simulink library "inp"  (R2021b)
settings: Solver=VariableStepAuto  StartTime=0.0  StopTime=10.0  RelTol=1e-3
undefined symbols (not defined in the file): C_TASK_5MS_S, FALSE, KINP_AcoreReadyToSlp_flg_ovrdflg, KINP_AcoreReadyToSlp_flg_ovrdval, KINP_AllowMovThd_OTA_enum_ovrdflg, KINP_AllowMovThd_OTA_enum_ovrdval, KINP_APSAngleTarget_Deg_ovrdflg, KINP_APSAngleTarget_Deg_ovrdval, KINP_APSDecReq_mps2_ovrdflg, KINP_APSDecReq_mps2_ovrdval, KINP_APSDecReqA_flg_ovrdflg, KINP_APSDecReqA_flg_ovrdval, KINP_APSDFLL_cm_ovrdflg, KINP_APSDFLL_cm_ovrdval, KINP_APSDFLR_cm_ovrdflg, KINP_APSDFLR_cm_ovrdval, KINP_APSDRLL_cm_ovrdflg, KINP_APSDRLL_cm_ovrdval, KINP_APSDRLR_cm_ovrdflg, KINP_APSDRLR_cm_ovrdval, KINP_APSExitCondition_enum_ovrdflg, KINP_APSExitCondition_enum_ovrdval, KINP_APSHWVer_enum_ovrdflg, KINP_APSHWVer_enum_ovrdval, KINP_APSProgressPCT_pct_ovrdflg, KINP_APSProgressPCT_pct_ovrdval, KINP_APSReq_enum_ovrdflg, KINP_APSReq_enum_ovrdval, KINP_APSRQDisplay_enum_ovrdflg, KINP_APSRQDisplay_enum_ovrdval, KINP_APSRqEPASCtrl_flg_ovrdflg, KINP_APSRqEPASCtrl_flg_ovrdval, KINP_APSShiftPosnReq_enum_ovrdval, KINP_APSShiftPosnReq_enum_ovrflg, KINP_APSSpeedCMD_kph_ovrdval, KINP_APSSpeedCMD_kph_ovrflg, KINP_APSStaSystem_enum_ovrdflg, KINP_APSStaSystem_enum_ovrdval, KINP_APSSWVer_enum_ovrdflg, KINP_APSSWVer_enum_ovrdval, KINP_APSVMCReqA_flg_ovrdval, KINP_APSVMCReqA_flg_ovrflg, KINP_APSVRqEPASCtrl_flg_ovrdflg, KINP_APSVRqEPASCtrl_flg_ovrdval, KINP_AuxBattVolmV_mV_ovrdflg, KINP_AuxBattVolmV_mV_ovrdval, KINP_CAASSta_enum_ovrdflg, KINP_CAASSta_enum_ovrdval, KINP_CAASVMCReqA_flg_ovrdval, KINP_CAASVMCReqA_flg_ovrflg, KINP_Chime_enum_ovrdflg, KINP_Chime_enum_ovrdval, KINP_ClearDTCcmd_flg_ovrdflg, KINP_ClearDTCcmd_flg_ovrdval, KINP_EvccAplusPwrUpReq_flg_ovrdflg, KINP_EvccAplusPwrUpReq_flg_ovrdval, KINP_LFID_raw_ovrdval, KINP_LFID_raw_ovrflg, KINP_LRID_raw_ovrdval, KINP_MemOffsetAccX_raw16_ovrdflg ... (+118)
libraries: FVT_lib x503, hcu_lib x1
(part 3 of 16)

== system inp/INP/CAN1/CommunicationCheck ==
  BHAL_outputs : Inport
  CANMsgInvalidDCDCStatus1 : FVT_lib/inp/CAN_Msg_Validity_Process_template  SystemSampleTime=-1  VariantActivationTime=update diagram  Latency=0  AutoFrameSizeCalculation=off
      link override ovrdflg: Value=KINP_CANMsgInvalidDCDCStatus1_flg_ovrdflg
      link override ovrdval: Value=KINP_CANMsgInvalidDCDCStatus1_flg_ovrdval
  CANMsgInvalidDCDCStatus2 : FVT_lib/inp/CAN_Msg_Validity_Process_template  SystemSampleTime=-1  VariantActivationTime=update diagram  Latency=0  AutoFrameSizeCalculation=off
      link override ovrdflg: Value=KINP_CANMsgInvalidDCDCStatus2_flg_ovrdflg
      link override ovrdval: Value=KINP_CANMsgInvalidDCDCStatus2_flg_ovrdval
  CANMsgInvalidEACStatus1 : FVT_lib/inp/CAN_Msg_Validity_Process_template  SystemSampleTime=-1  VariantActivationTime=update diagram  Latency=0  AutoFrameSizeCalculation=off
      link override ovrdflg: Value=KINP_CANMsgInvalidEACStatus1_flg_ovrdflg
      link override ovrdval: Value=KINP_CANMsgInvalidEACStatus1_flg_ovrdval
  CANMsgInvalidEBC1 : FVT_lib/inp/CAN_Msg_Validity_Process_template  SystemSampleTime=-1  VariantActivationTime=update diagram  Latency=0  AutoFrameSizeCalculation=off
      link override ovrdflg: Value=KINP_CANMsgInvalidEBC1_flg_ovrdflg
      link override ovrdval: Value=KINP_CANMsgInvalidEBC1_flg_ovrdval
  CANMsgInvalidEBC2 : FVT_lib/inp/CAN_Msg_Validity_Process_template  SystemSampleTime=-1  VariantActivationTime=update diagram  Latency=0  AutoFrameSizeCalculation=off
      link override ovrdflg: Value=KINP_CANMsgInvalidEBC2_flg_ovrdflg
      link override ovrdval: Value=KINP_CANMsgInvalidEBC2_flg_ovrdval
  CANMsgInvalidEBC5 : FVT_lib/inp/CAN_Msg_Validity_Process_template  SystemSampleTime=-1  VariantActivationTime=update diagram  Latency=0  AutoFrameSizeCalculation=off
      link override ovrdflg: Value=KINP_CANMsgInvalidEBC5_flg_ovrdflg
      link override ovrdval: Value=KINP_CANMsgInvalidEBC5_flg_ovrdval
  CANMsgInvalidEHPSStatus1 : FVT_lib/inp/CAN_Msg_Validity_Process_template  SystemSampleTime=-1  VariantActivationTime=update diagram  Latency=0  AutoFrameSizeCalculation=off
      link override ovrdflg: Value=KINP_CANMsgInvalidEHPSStatus1_flg_ovrdflg
      link override ovrdval: Value=KINP_CANMsgInvalidEHPSStatus1_flg_ovrdval
  CANMsgInvalidEMC1EM1 : FVT_lib/inp/CAN_Msg_Validity_Process_template  SystemSampleTime=-1  VariantActivationTime=update diagram  Latency=0  AutoFrameSizeCalculation=off
      link override ovrdflg: Value=KINP_CANMsgInvalidEMC1EM1_flg_ovrdflg
      link override ovrdval: Value=KINP_CANMsgInvalidEMC1EM1_flg_ovrdval
  CANMsgInvalidEPB1 : FVT_lib/inp/CAN_Msg_Validity_Process_template  SystemSampleTime=-1  VariantActivationTime=update diagram  Latency=0  AutoFrameSizeCalculation=off
      link override ovrdflg: Value=KINP_CANMsgInvalidEPB1_flg_ovrdflg
      link override ovrdval: Value=KINP_CANMsgInvalidEPB1_flg_ovrdval
  CANMsgInvalidPDUStatus1 : FVT_lib/inp/CAN_Msg_Validity_Process_template  SystemSampleTime=-1  VariantActivationTime=update diagram  Latency=0  AutoFrameSizeCalculation=off
      link override ovrdflg: Value=KINP_CANMsgInvalidPDUStatus1_flg_ovrdflg
      link override ovrdval: Value=KINP_CANMsgInvalidPDUStatus1_flg_ovrdval
  bus_creator : BusCreator  Inputs=10
  bus_selector : BusSelector  OutputSignals=VHAL_CANMsgInvalidDCDCStatus1_flg,VHAL_CANMsgInvalidDCDCStatus2_flg,VHAL_CANMsgInvalidEACStatus1_flg,VHAL_CANMsgInvalidEBC1_flg,VHAL_CANMsgInvalidEBC2_flg,VHAL_CANMsgInvalidEBC5_flg,VHAL_CANMsgInvalidEHPSStatus1_flg,VHAL_CANMsgInvalidEMC1EM1_flg,VHAL_CANMsgInvalidEPB1_flg,VHAL_CANMsgInvalidPDUStatus1_flg
  not{1..10} (10 alike) : Logic  Operator=NOT  AllPortsSameDT=off  OutDataTypeStr=boolean
  inp_CanValid_bus : Outport
  wires:
  BHAL_outputs/1 -> [BHAL_outputs]
  bus_selector/1 -> CANMsgInvalidDCDCStatus1/1  "<VHAL_CANMsgInvalidDCDCStatus1_flg>"
  CANMsgInvalidDCDCStatus1/1 -> not1/1
  not1/1 -> bus_creator/1  "VINP_CANMsgValidDCDCStatus1_flg"
  bus_selector/2 -> CANMsgInvalidDCDCStatus2/1  "<VHAL_CANMsgInvalidDCDCStatus2_flg>"
  CANMsgInvalidDCDCStatus2/1 -> not2/1
  not2/1 -> bus_creator/2  "VINP_CANMsgValidDCDCStatus2_flg"
  bus_selector/3 -> CANMsgInvalidEACStatus1/1  "<VHAL_CANMsgInvalidEACStatus1_flg>"
  CANMsgInvalidEACStatus1/1 -> not3/1
  not3/1 -> bus_creator/3  "VINP_CANMsgValidEACStatus1_flg"
  bus_selector/4 -> CANMsgInvalidEBC1/1  "<VHAL_CANMsgInvalidEBC1_flg>"
  CANMsgInvalidEBC1/1 -> not4/1
  not4/1 -> bus_creator/4  "VINP_CANMsgValidEBC1_flg"
  bus_selector/5 -> CANMsgInvalidEBC2/1  "<VHAL_CANMsgInvalidEBC2_flg>"
  CANMsgInvalidEBC2/1 -> not5/1
  not5/1 -> bus_creator/5  "VINP_CANMsgValidEBC2_flg"
  bus_selector/6 -> CANMsgInvalidEBC5/1  "<VHAL_CANMsgInvalidEBC5_flg>"
  CANMsgInvalidEBC5/1 -> not6/1
  not6/1 -> bus_creator/6  "VINP_CANMsgValidEBC5_flg"
  bus_selector/7 -> CANMsgInvalidEHPSStatus1/1  "<VHAL_CANMsgInvalidEHPSStatus1_flg>"
  CANMsgInvalidEHPSStatus1/1 -> not7/1
  not7/1 -> bus_creator/7  "VINP_CANMsgValidEHPSStatus1_flg"
  bus_selector/8 -> CANMsgInvalidEMC1EM1/1  "<VHAL_CANMsgInvalidEMC1EM1_flg>"
  CANMsgInvalidEMC1EM1/1 -> not8/1
  not8/1 -> bus_creator/8  "VINP_CANMsgValidEMC1EM1_flg"
  bus_selector/9 -> CANMsgInvalidEPB1/1  "<VHAL_CANMsgInvalidEPB1_flg>"
  CANMsgInvalidEPB1/1 -> not9/1
  not9/1 -> bus_creator/9  "VINP_CANMsgValidEPB1_flg"
  bus_selector/10 -> CANMsgInvalidPDUStatus1/1  "<VHAL_CANMsgInvalidPDUStatus1_flg>"
  CANMsgInvalidPDUStatus1/1 -> not10/1
  not10/1 -> bus_creator/10  "VINP_CANMsgValidPDUStatus1_flg"
  [BHAL_outputs] -> bus_selector/1
  bus_creator/1 -> inp_CanValid_bus/1

== system inp/INP/CAN1/CreateBus ==
  inp_CanValid_bus : Inport
  inp_Hal_bus : Inport  Port=2
  UnitConverter_{1..10} (10 alike) : DataTypeConversion  OutDataTypeStr=boolean
  UnitConverter_{11,13..22,24..28,30..31,33..35,39..43,45..53,58..62} (40 alike) : DataTypeConversion  OutDataTypeStr=uint8
  UnitConverter_{12,23,29,32,36..38,44,54..57} (12 alike) : DataTypeConversion  OutDataTypeStr=single
  bus_creator : BusCreator  Inputs=62
  bus_selector : BusSelector  OutputSignals=VINP_CANMsgValidDCDCStatus1_flg,VINP_CANMsgValidDCDCStatus2_flg,VINP_CANMsgValidEACStatus1_flg,VINP_CANMsgValidEBC1_flg,VINP_CANMsgValidEBC2_flg,VINP_CANMsgValidEBC5_flg,VINP_CANMsgValidEHPSStatus1_flg,VINP_CANMsgValidEMC1EM1_flg,VINP_CANMsgValidEPB1_flg,VINP_CANMsgValidPDUStatus1_flg
  bus_selector_1 : BusSelector  OutputSignals=VINP_DCDCEnSta_enum,VINP_DCDCOutVol_V,VINP_EACEnSta_enum,VINP_ABSFullyOper_enum,VINP_ABSOffroadSw_enum,VINP_ASRBrakeCtrlAtc_enum,VINP_ASREngCtrlAtc_enum,VINP_ASRHillHolderSw_enum,VINP_ASROffroadSw_enum,VINP_ATCASRInfoSig_enum,VINP_AcltrInterlockSw_enum,VINP_AntiLBrakABSAct_enum,VINP_BrakePedalPos_pct,VINP_EBSAmWarnLampSta_enum,VINP_EBSBrakeSw_enum,VINP_EBSRedWarnLampSta_enum,VINP_EngAuxShutdownSw_enum,VINP_EngDerateSw_enum,VINP_EngRetSel_pct,VINP_HaltBrakeSw_enum,VINP_RmAccelEnSw_enum,VINP_SACtrlBrakeCtrl_SA,VINP_TractCtrlOvrSw_enum,VINP_TrailerABSSta_enum,VINP_TrailerABSWarnSig_enum,VINP_FASpeed_kph,VINP_RelaSpdFALWheel_kph,VINP_RelaSpdFARWheel_kph,VINP_BrkTempeWarn_enum,VINP_FndBrkUse_enum,VINP_HaltBrkMode_enum,VINP_HillHolderMode_enum,VINP_ParkBrkActuFAct_enum,VINP_XBRAcltnLimit_mps2,VINP_XBRActtrlMode_enum,VINP_XBRSysSta_enum,VINP_EHPSEnSta_enum,VINP_EM1CS_enum,VINP_EM1Cnt_enum,VINP_EM1OvrCtrlMBrk_enum,VINP_EM1OvrCtrlMDriv_enum,VINP_EM1OvrCtrlMPriBrk_enum,VINP_EM1OvrCtrlMPriDriv_enum,VINP_EM1ReqTorqHRlsBrk_pct,VINP_EM1ReqTorqHRlsDri_pct,VINP_EM1ReqTorqLimBrk_pct,VINP_EM1ReqTorqLimDriv_pct,VINP_EPBParkingBrakeSta_enum,VINP_PDUDCDCRlySta_enum,VINP_PDUEACRlySta_enum,VINP_PDUEHPSRlySta_enum,VINP_PDUSelfChkSta_enum
  BINP_outputs : Outport
  wires:
  inp_CanValid_bus/1 -> [inp_CanValid_bus]
  inp_Hal_bus/1 -> [inp_Hal_bus]
  bus_selector/1 -> UnitConverter_1/1  "<VINP_CANMsgValidDCDCStatus1_flg>"
  UnitConverter_1/1 -> bus_creator/1  "VINP_CANMsgValidDCDCStatus1_flg"
  bus_selector/2 -> UnitConverter_2/1  "<VINP_CANMsgValidDCDCStatus2_flg>"
  UnitConverter_2/1 -> bus_creator/2  "VINP_CANMsgValidDCDCStatus2_flg"
  bus_selector/3 -> UnitConverter_3/1  "<VINP_CANMsgValidEACStatus1_flg>"
  UnitConverter_3/1 -> bus_creator/3  "VINP_CANMsgValidEACStatus1_flg"
  bus_selector/4 -> UnitConverter_4/1  "<VINP_CANMsgValidEBC1_flg>"
  UnitConverter_4/1 -> bus_creator/4  "VINP_CANMsgValidEBC1_flg"
  bus_selector/5 -> UnitConverter_5/1  "<VINP_CANMsgValidEBC2_flg>"
  UnitConverter_5/1 -> bus_creator/5  "VINP_CANMsgValidEBC2_flg"
  bus_selector/6 -> UnitConverter_6/1  "<VINP_CANMsgValidEBC5_flg>"
  UnitConverter_6/1 -> bus_creator/6  "VINP_CANMsgValidEBC5_flg"
  bus_selector/7 -> UnitConverter_7/1  "<VINP_CANMsgValidEHPSStatus1_flg>"
  UnitConverter_7/1 -> bus_creator/7  "VINP_CANMsgValidEHPSStatus1_flg"
  bus_selector/8 -> UnitConverter_8/1  "<VINP_CANMsgValidEMC1EM1_flg>"
  UnitConverter_8/1 -> bus_creator/8  "VINP_CANMsgValidEMC1EM1_flg"
  bus_selector/9 -> UnitConverter_9/1  "<VINP_CANMsgValidEPB1_flg>"
  UnitConverter_9/1 -> bus_creator/9  "VINP_CANMsgValidEPB1_flg"
  bus_selector/10 -> UnitConverter_10/1  "<VINP_CANMsgValidPDUStatus1_flg>"
  UnitConverter_10/1 -> bus_creator/10  "VINP_CANMsgValidPDUStatus1_flg"
  bus_selector_1/1 -> UnitConverter_11/1  "<VINP_DCDCEnSta_enum>"
  UnitConverter_11/1 -> bus_creator/11  "VINP_DCDCEnSta_enum"
  bus_selector_1/2 -> UnitConverter_12/1  "<VINP_DCDCOutVol_V>"
  UnitConverter_12/1 -> bus_creator/12  "VINP_DCDCOutVol_V"
  bus_selector_1/3 -> UnitConverter_13/1  "<VINP_EACEnSta_enum>"
  UnitConverter_13/1 -> bus_creator/13  "VINP_EACEnSta_enum"
  bus_selector_1/4 -> UnitConverter_14/1  "<VINP_ABSFullyOper_enum>"
  UnitConverter_14/1 -> bus_creator/14  "VINP_ABSFullyOper_enum"
  bus_selector_1/5 -> UnitConverter_15/1  "<VINP_ABSOffroadSw_enum>"
  UnitConverter_15/1 -> bus_creator/15  "VINP_ABSOffroadSw_enum"
  bus_selector_1/6 -> UnitConverter_16/1  "<VINP_ASRBrakeCtrlAtc_enum>"
  UnitConverter_16/1 -> bus_creator/16  "VINP_ASRBrakeCtrlAtc_enum"
  bus_selector_1/7 -> UnitConverter_17/1  "<VINP_ASREngCtrlAtc_enum>"
  UnitConverter_17/1 -> bus_creator/17  "VINP_ASREngCtrlAtc_enum"
  bus_selector_1/8 -> UnitConverter_18/1  "<VINP_ASRHillHolderSw_enum>"
  UnitConverter_18/1 -> bus_creator/18  "VINP_ASRHillHolderSw_enum"
  bus_selector_1/9 -> UnitConverter_19/1  "<VINP_ASROffroadSw_enum>"
  UnitConverter_19/1 -> bus_creator/19  "VINP_ASROffroadSw_enum"
  bus_selector_1/10 -> UnitConverter_20/1  "<VINP_ATCASRInfoSig_enum>"
  UnitConverter_20/1 -> bus_creator/20  "VINP_ATCASRInfoSig_enum"
  bus_selector_1/11 -> UnitConverter_21/1  "<VINP_AcltrInterlockSw_enum>"
  UnitConverter_21/1 -> bus_creator/21  "VINP_AcltrInterlockSw_enum"
  bus_selector_1/12 -> UnitConverter_22/1  "<VINP_AntiLBrakABSAct_enum>"
  UnitConverter_22/1 -> bus_creator/22  "VINP_AntiLBrakABSAct_enum"
  bus_selector_1/13 -> UnitConverter_23/1  "<VINP_BrakePedalPos_pct>"
  UnitConverter_23/1 -> bus_creator/23  "VINP_BrakePedalPos_pct"
  bus_selector_1/14 -> UnitConverter_24/1  "<VINP_EBSAmWarnLampSta_enum>"
  UnitConverter_24/1 -> bus_creator/24  "VINP_EBSAmWarnLampSta_enum"
  bus_selector_1/15 -> UnitConverter_25/1  "<VINP_EBSBrakeSw_enum>"
  UnitConverter_25/1 -> bus_creator/25  "VINP_EBSBrakeSw_enum"
  bus_selector_1/16 -> UnitConverter_26/1  "<VINP_EBSRedWarnLampSta_enum>"
  UnitConverter_26/1 -> bus_creator/26  "VINP_EBSRedWarnLampSta_enum"
  bus_selector_1/17 -> UnitConverter_27/1  "<VINP_EngAuxShutdownSw_enum>"
  UnitConverter_27/1 -> bus_creator/27  "VINP_EngAuxShutdownSw_enum"
  bus_selector_1/18 -> UnitConverter_28/1  "<VINP_EngDerateSw_enum>"
  UnitConverter_28/1 -> bus_creator/28  "VINP_EngDerateSw_enum"
  bus_selector_1/19 -> UnitConverter_29/1  "<VINP_EngRetSel_pct>"
  UnitConverter_29/1 -> bus_creator/29  "VINP_EngRetSel_pct"
  bus_selector_1/20 -> UnitConverter_30/1  "<VINP_HaltBrakeSw_enum>"
  UnitConverter_30/1 -> bus_creator/30  "VINP_HaltBrakeSw_enum"
  bus_selector_1/21 -> UnitConverter_31/1  "<VINP_RmAccelEnSw_enum>"
  UnitConverter_31/1 -> bus_creator/31  "VINP_RmAccelEnSw_enum"
  bus_selector_1/22 -> UnitConverter_32/1  "<VINP_SACtrlBrakeCtrl_SA>"
  UnitConverter_32/1 -> bus_creator/32  "VINP_SACtrlBrakeCtrl_SA"
  bus_selector_1/23 -> UnitConverter_33/1  "<VINP_TractCtrlOvrSw_enum>"
  UnitConverter_33/1 -> bus_creator/33  "VINP_TractCtrlOvrSw_enum"
  bus_selector_1/24 -> UnitConverter_34/1  "<VINP_TrailerABSSta_enum>"
  UnitConverter_34/1 -> bus_creator/34  "VINP_TrailerABSSta_enum"
  bus_selector_1/25 -> UnitConverter_35/1  "<VINP_TrailerABSWarnSig_enum>"
  UnitConverter_35/1 -> bus_creator/35  "VINP_TrailerABSWarnSig_enum"
  bus_selector_1/26 -> UnitConverter_36/1  "<VINP_FASpeed_kph>"
  UnitConverter_36/1 -> bus_creator/36  "VINP_FASpeed_kph"
  bus_selector_1/27 -> UnitConverter_37/1  "<VINP_RelaSpdFALWheel_kph>"
  UnitConverter_37/1 -> bus_creator/37  "VINP_RelaSpdFALWheel_kph"
  bus_selector_1/28 -> UnitConverter_38/1  "<VINP_RelaSpdFARWheel_kph>"
  UnitConverter_38/1 -> bus_creator/38  "VINP_RelaSpdFARWheel_kph"
  bus_selector_1/29 -> UnitConverter_39/1  "<VINP_BrkTempeWarn_enum>"
  UnitConverter_39/1 -> bus_creator/39  "VINP_BrkTempeWarn_enum"
  bus_selector_1/30 -> UnitConverter_40/1  "<VINP_FndBrkUse_enum>"
  UnitConverter_40/1 -> bus_creator/40  "VINP_FndBrkUse_enum"
  bus_selector_1/31 -> UnitConverter_41/1  "<VINP_HaltBrkMode_enum>"
  UnitConverter_41/1 -> bus_creator/41  "VINP_HaltBrkMode_enum"
  bus_selector_1/32 -> UnitConverter_42/1  "<VINP_HillHolderMode_enum>"
  UnitConverter_42/1 -> bus_creator/42  "VINP_HillHolderMode_enum"
  bus_selector_1/33 -> UnitConverter_43/1  "<VINP_ParkBrkActuFAct_enum>"
  UnitConverter_43/1 -> bus_creator/43  "VINP_ParkBrkActuFAct_enum"
  bus_selector_1/34 -> UnitConverter_44/1  "<VINP_XBRAcltnLimit_mps2>"
  UnitConverter_44/1 -> bus_creator/44  "VINP_XBRAcltnLimit_mps2"
  bus_selector_1/35 -> UnitConverter_45/1  "<VINP_XBRActtrlMode_enum>"
  UnitConverter_45/1 -> bus_creator/45  "VINP_XBRActtrlMode_enum"
  bus_selector_1/36 -> UnitConverter_46/1  "<VINP_XBRSysSta_enum>"
  UnitConverter_46/1 -> bus_creator/46  "VINP_XBRSysSta_enum"
  bus_selector_1/37 -> UnitConverter_47/1  "<VINP_EHPSEnSta_enum>"
  UnitConverter_47/1 -> bus_creator/47  "VINP_EHPSEnSta_enum"
  bus_selector_1/38 -> UnitConverter_48/1  "<VINP_EM1CS_enum>"
  UnitConverter_48/1 -> bus_creator/48  "VINP_EM1CS_enum"
  bus_selector_1/39 -> UnitConverter_49/1  "<VINP_EM1Cnt_enum>"
  UnitConverter_49/1 -> bus_creator/49  "VINP_EM1Cnt_enum"
  bus_selector_1/40 -> UnitConverter_50/1  "<VINP_EM1OvrCtrlMBrk_enum>"
  UnitConverter_50/1 -> bus_creator/50  "VINP_EM1OvrCtrlMBrk_enum"
  bus_selector_1/41 -> UnitConverter_51/1  "<VINP_EM1OvrCtrlMDriv_enum>"
  UnitConverter_51/1 -> bus_creator/51  "VINP_EM1OvrCtrlMDriv_enum"
  bus_selector_1/42 -> UnitConverter_52/1  "<VINP_EM1OvrCtrlMPriBrk_enum>"
  UnitConverter_52/1 -> bus_creator/52  "VINP_EM1OvrCtrlMPriBrk_enum"
  bus_selector_1/43 -> UnitConverter_53/1  "<VINP_EM1OvrCtrlMPriDriv_enum>"
  UnitConverter_53/1 -> bus_creator/53  "VINP_EM1OvrCtrlMPriDriv_enum"
  bus_selector_1/44 -> UnitConverter_54/1  "<VINP_EM1ReqTorqHRlsBrk_pct>"
  UnitConverter_54/1 -> bus_creator/54  "VINP_EM1ReqTorqHRlsBrk_pct"
  bus_selector_1/45 -> UnitConverter_55/1  "<VINP_EM1ReqTorqHRlsDri_pct>"
  UnitConverter_55/1 -> bus_creator/55  "VINP_EM1ReqTorqHRlsDri_pct"
  bus_selector_1/46 -> UnitConverter_56/1  "<VINP_EM1ReqTorqLimBrk_pct>"
  UnitConverter_56/1 -> bus_creator/56  "VINP_EM1ReqTorqLimBrk_pct"
  bus_selector_1/47 -> UnitConverter_57/1  "<VINP_EM1ReqTorqLimDriv_pct>"
  UnitConverter_57/1 -> bus_creator/57  "VINP_EM1ReqTorqLimDriv_pct"
  bus_selector_1/48 -> UnitConverter_58/1  "<VINP_EPBParkingBrakeSta_enum>"
  UnitConverter_58/1 -> bus_creator/58  "VINP_EPBParkingBrakeSta_enum"
  bus_selector_1/49 -> UnitConverter_59/1  "<VINP_PDUDCDCRlySta_enum>"
  UnitConverter_59/1 -> bus_creator/59  "VINP_PDUDCDCRlySta_enum"
  bus_selector_1/50 -> UnitConverter_60/1  "<VINP_PDUEACRlySta_enum>"
  UnitConverter_60/1 -> bus_creator/60  "VINP_PDUEACRlySta_enum"
  bus_selector_1/51 -> UnitConverter_61/1  "<VINP_PDUEHPSRlySta_enum>"
  UnitConverter_61/1 -> bus_creator/61  "VINP_PDUEHPSRlySta_enum"
  bus_selector_1/52 -> UnitConverter_62/1  "<VINP_PDUSelfChkSta_enum>"
  UnitConverter_62/1 -> bus_creator/62  "VINP_PDUSelfChkSta_enum"
  [inp_CanValid_bus] -> bus_selector/1
  [inp_Hal_bus] -> bus_selector_1/1
  bus_creator/1 -> BINP_outputs/1

== system inp/INP/CAN1/SignalCheck ==
  inp_CanValid_bus : Inport
  TASK_TIME_S : Inport  Port=2
  BHAL_outputs : Inport  Port=3
  DCDC_Status_1 : Subsystem
  DCDC_Status_2 : Subsystem
  EAC_Status_1 : Subsystem
  EBC1 : Subsystem
  EBC2 : Subsystem
  EBC5 : Subsystem
  EHPS_Status_1 : Subsystem
  EMC1_EM1 : Subsystem
  EPB1 : Subsystem
  PDU_Status_1 : Subsystem
  bus_creator : BusCreator  Inputs=52
  inp_Hal_bus : Outport
  wires:
  inp_CanValid_bus/1 -> [inp_CanValid_bus]
  TASK_TIME_S/1 -> [TASK_TIME_S]
  BHAL_outputs/1 -> [BHAL_outputs]
  [BHAL_outputs] -> DCDC_Status_1/1(BHAL_outputs)
  [inp_CanValid_bus] -> DCDC_Status_1/2(inp_CanValid_bus)
  DCDC_Status_1/1(VINP_DCDCEnSta_enum) -> [VINP_DCDCEnSta_enum]
  [BHAL_outputs] -> DCDC_Status_2/1(BHAL_outputs)
  [inp_CanValid_bus] -> DCDC_Status_2/2(inp_CanValid_bus)
  DCDC_Status_2/1(VINP_DCDCOutVol_V) -> [VINP_DCDCOutVol_V]
  [BHAL_outputs] -> EAC_Status_1/1(BHAL_outputs)
  [inp_CanValid_bus] -> EAC_Status_1/2(inp_CanValid_bus)
  EAC_Status_1/1(VINP_EACEnSta_enum) -> [VINP_EACEnSta_enum]
  [BHAL_outputs] -> EBC1/1(BHAL_outputs)
  [inp_CanValid_bus] -> EBC1/2(inp_CanValid_bus)
  EBC1/1(VINP_ABSFullyOper_enum) -> [VINP_ABSFullyOper_enum]
  EBC1/2(VINP_ABSOffroadSw_enum) -> [VINP_ABSOffroadSw_enum]
  EBC1/3(VINP_ASRBrakeCtrlAtc_enum) -> [VINP_ASRBrakeCtrlAtc_enum]
  EBC1/4(VINP_ASREngCtrlAtc_enum) -> [VINP_ASREngCtrlAtc_enum]
  EBC1/5(VINP_ASRHillHolderSw_enum) -> [VINP_ASRHillHolderSw_enum]
  EBC1/6(VINP_ASROffroadSw_enum) -> [VINP_ASROffroadSw_enum]
  EBC1/7(VINP_ATCASRInfoSig_enum) -> [VINP_ATCASRInfoSig_enum]
  EBC1/8(VINP_AcltrInterlockSw_enum) -> [VINP_AcltrInterlockSw_enum]
  EBC1/9(VINP_AntiLBrakABSAct_enum) -> [VINP_AntiLBrakABSAct_enum]
  EBC1/10(VINP_BrakePedalPos_pct) -> [VINP_BrakePedalPos_pct]
  EBC1/11(VINP_EBSAmWarnLampSta_enum) -> [VINP_EBSAmWarnLampSta_enum]
  EBC1/12(VINP_EBSBrakeSw_enum) -> [VINP_EBSBrakeSw_enum]
  EBC1/13(VINP_EBSRedWarnLampSta_enum) -> [VINP_EBSRedWarnLampSta_enum]
  EBC1/14(VINP_EngAuxShutdownSw_enum) -> [VINP_EngAuxShutdownSw_enum]
  EBC1/15(VINP_EngDerateSw_enum) -> [VINP_EngDerateSw_enum]
  EBC1/16(VINP_EngRetSel_pct) -> [VINP_EngRetSel_pct]
  EBC1/17(VINP_HaltBrakeSw_enum) -> [VINP_HaltBrakeSw_enum]
  EBC1/18(VINP_RmAccelEnSw_enum) -> [VINP_RmAccelEnSw_enum]
  EBC1/19(VINP_SACtrlBrakeCtrl_SA) -> [VINP_SACtrlBrakeCtrl_SA]
  EBC1/20(VINP_TractCtrlOvrSw_enum) -> [VINP_TractCtrlOvrSw_enum]
  EBC1/21(VINP_TrailerABSSta_enum) -> [VINP_TrailerABSSta_enum]
  EBC1/22(VINP_TrailerABSWarnSig_enum) -> [VINP_TrailerABSWarnSig_enum]
  [BHAL_outputs] -> EBC2/1(BHAL_outputs)
  [inp_CanValid_bus] -> EBC2/2(inp_CanValid_bus)
  EBC2/1(VINP_FASpeed_kph) -> [VINP_FASpeed_kph]
  EBC2/2(VINP_RelaSpdFALWheel_kph) -> [VINP_RelaSpdFALWheel_kph]
  EBC2/3(VINP_RelaSpdFARWheel_kph) -> [VINP_RelaSpdFARWheel_kph]
  [BHAL_outputs] -> EBC5/1(BHAL_outputs)
  [inp_CanValid_bus] -> EBC5/2(inp_CanValid_bus)
  EBC5/1(VINP_BrkTempeWarn_enum) -> [VINP_BrkTempeWarn_enum]
  EBC5/2(VINP_FndBrkUse_enum) -> [VINP_FndBrkUse_enum]
  EBC5/3(VINP_HaltBrkMode_enum) -> [VINP_HaltBrkMode_enum]
  EBC5/4(VINP_HillHolderMode_enum) -> [VINP_HillHolderMode_enum]
  EBC5/5(VINP_ParkBrkActuFAct_enum) -> [VINP_ParkBrkActuFAct_enum]
  EBC5/6(VINP_XBRAcltnLimit_mps2) -> [VINP_XBRAcltnLimit_mps2]
  EBC5/7(VINP_XBRActtrlMode_enum) -> [VINP_XBRActtrlMode_enum]
  EBC5/8(VINP_XBRSysSta_enum) -> [VINP_XBRSysSta_enum]
  [BHAL_outputs] -> EHPS_Status_1/1(BHAL_outputs)
  [inp_CanValid_bus] -> EHPS_Status_1/2(inp_CanValid_bus)
  EHPS_Status_1/1(VINP_EHPSEnSta_enum) -> [VINP_EHPSEnSta_enum]
  [BHAL_outputs] -> EMC1_EM1/1(BHAL_outputs)
  [inp_CanValid_bus] -> EMC1_EM1/2(inp_CanValid_bus)
  EMC1_EM1/1(VINP_EM1CS_enum) -> [VINP_EM1CS_enum]
  EMC1_EM1/2(VINP_EM1Cnt_enum) -> [VINP_EM1Cnt_enum]
  EMC1_EM1/3(VINP_EM1OvrCtrlMBrk_enum) -> [VINP_EM1OvrCtrlMBrk_enum]
  EMC1_EM1/4(VINP_EM1OvrCtrlMDriv_enum) -> [VINP_EM1OvrCtrlMDriv_enum]
  EMC1_EM1/5(VINP_EM1OvrCtrlMPriBrk_enum) -> [VINP_EM1OvrCtrlMPriBrk_enum]
  EMC1_EM1/6(VINP_EM1OvrCtrlMPriDriv_enum) -> [VINP_EM1OvrCtrlMPriDriv_enum]
  EMC1_EM1/7(VINP_EM1ReqTorqHRlsBrk_pct) -> [VINP_EM1ReqTorqHRlsBrk_pct]
  EMC1_EM1/8(VINP_EM1ReqTorqHRlsDri_pct) -> [VINP_EM1ReqTorqHRlsDri_pct]
  EMC1_EM1/9(VINP_EM1ReqTorqLimBrk_pct) -> [VINP_EM1ReqTorqLimBrk_pct]
  EMC1_EM1/10(VINP_EM1ReqTorqLimDriv_pct) -> [VINP_EM1ReqTorqLimDriv_pct]
  [BHAL_outputs] -> EPB1/1(BHAL_outputs)
  [inp_CanValid_bus] -> EPB1/2(inp_CanValid_bus)
  EPB1/1(VINP_EPBParkingBrakeSta_enum) -> [VINP_EPBParkingBrakeSta_enum]
  [BHAL_outputs] -> PDU_Status_1/1(BHAL_outputs)
  [inp_CanValid_bus] -> PDU_Status_1/2(inp_CanValid_bus)
  PDU_Status_1/1(VINP_PDUDCDCRlySta_enum) -> [VINP_PDUDCDCRlySta_enum]
  PDU_Status_1/2(VINP_PDUEACRlySta_enum) -> [VINP_PDUEACRlySta_enum]
  PDU_Status_1/3(VINP_PDUEHPSRlySta_enum) -> [VINP_PDUEHPSRlySta_enum]
  PDU_Status_1/4(VINP_PDUSelfChkSta_enum) -> [VINP_PDUSelfChkSta_enum]
  bus_creator/1 -> inp_Hal_bus/1
  [VINP_DCDCEnSta_enum] -> bus_creator/1
  [VINP_DCDCOutVol_V] -> bus_creator/2
  [VINP_EACEnSta_enum] -> bus_creator/3
  [VINP_ABSFullyOper_enum] -> bus_creator/4
  [VINP_ABSOffroadSw_enum] -> bus_creator/5
  [VINP_ASRBrakeCtrlAtc_enum] -> bus_creator/6
  [VINP_ASREngCtrlAtc_enum] -> bus_creator/7
  [VINP_ASRHillHolderSw_enum] -> bus_creator/8
  [VINP_ASROffroadSw_enum] -> bus_creator/9
  [VINP_ATCASRInfoSig_enum] -> bus_creator/10
  [VINP_AcltrInterlockSw_enum] -> bus_creator/11
  [VINP_AntiLBrakABSAct_enum] -> bus_creator/12
  [VINP_BrakePedalPos_pct] -> bus_creator/13
  [VINP_EBSAmWarnLampSta_enum] -> bus_creator/14
  [VINP_EBSBrakeSw_enum] -> bus_creator/15
  [VINP_EBSRedWarnLampSta_enum] -> bus_creator/16
  [VINP_EngAuxShutdownSw_enum] -> bus_creator/17
  [VINP_EngDerateSw_enum] -> bus_creator/18
  [VINP_EngRetSel_pct] -> bus_creator/19
  [VINP_HaltBrakeSw_enum] -> bus_creator/20
  [VINP_RmAccelEnSw_enum] -> bus_creator/21
  [VINP_SACtrlBrakeCtrl_SA] -> bus_creator/22
  [VINP_TractCtrlOvrSw_enum] -> bus_creator/23
  [VINP_TrailerABSSta_enum] -> bus_creator/24
  [VINP_TrailerABSWarnSig_enum] -> bus_creator/25
  [VINP_FASpeed_kph] -> bus_creator/26
  [VINP_RelaSpdFALWheel_kph] -> bus_creator/27
  [VINP_RelaSpdFARWheel_kph] -> bus_creator/28
  [VINP_BrkTempeWarn_enum] -> bus_creator/29
  [VINP_FndBrkUse_enum] -> bus_creator/30
  [VINP_HaltBrkMode_enum] -> bus_creator/31
  [VINP_HillHolderMode_enum] -> bus_creator/32
  [VINP_ParkBrkActuFAct_enum] -> bus_creator/33
  [VINP_XBRAcltnLimit_mps2] -> bus_creator/34
  [VINP_XBRActtrlMode_enum] -> bus_creator/35
  [VINP_XBRSysSta_enum] -> bus_creator/36
  [VINP_EHPSEnSta_enum] -> bus_creator/37
  [VINP_EM1CS_enum] -> bus_creator/38
  [VINP_EM1Cnt_enum] -> bus_creator/39
  [VINP_EM1OvrCtrlMBrk_enum] -> bus_creator/40
  [VINP_EM1OvrCtrlMDriv_enum] -> bus_creator/41
  [VINP_EM1OvrCtrlMPriBrk_enum] -> bus_creator/42
  [VINP_EM1OvrCtrlMPriDriv_enum] -> bus_creator/43
  [VINP_EM1ReqTorqHRlsBrk_pct] -> bus_creator/44
  [VINP_EM1ReqTorqHRlsDri_pct] -> bus_creator/45
  [VINP_EM1ReqTorqLimBrk_pct] -> bus_creator/46
  [VINP_EM1ReqTorqLimDriv_pct] -> bus_creator/47
  [VINP_EPBParkingBrakeSta_enum] -> bus_creator/48
  [VINP_PDUDCDCRlySta_enum] -> bus_creator/49
  [VINP_PDUEACRlySta_enum] -> bus_creator/50
  [VINP_PDUEHPSRlySta_enum] -> bus_creator/51
  [VINP_PDUSelfChkSta_enum] -> bus_creator/52

== system inp/INP/CAN2/CommunicationCheck ==
  BHAL_outputs : Inport
  CANMsgInvalidIVI1 : FVT_lib/inp/CAN_Msg_Validity_Process_template  SystemSampleTime=-1  VariantActivationTime=update diagram  Latency=0  AutoFrameSizeCalculation=off
      link override ovrdflg: Value=KINP_CANMsgInvalidIVI1_flg_ovrdflg
      link override ovrdval: Value=KINP_CANMsgInvalidIVI1_flg_ovrdval
  CANMsgInvalidIVI2 : FVT_lib/inp/CAN_Msg_Validity_Process_template  SystemSampleTime=-1  VariantActivationTime=update diagram  Latency=0  AutoFrameSizeCalculation=off
      link override ovrdflg: Value=KINP_CANMsgInvalidIVI2_flg_ovrdflg
      link override ovrdval: Value=KINP_CANMsgInvalidIVI2_flg_ovrdval
  CANMsgInvalidIVIP200 : FVT_lib/inp/CAN_Msg_Validity_Process_template  SystemSampleTime=-1  VariantActivationTime=update diagram  Latency=0  AutoFrameSizeCalculation=off
      link override ovrdflg: Value=KINP_CANMsgInvalidIVIP200_flg_ovrdflg
      link override ovrdval: Value=KINP_CANMsgInvalidIVIP200_flg_ovrdval
  CANMsgInvalidMETER1 : FVT_lib/inp/CAN_Msg_Validity_Process_template  SystemSampleTime=-1  VariantActivationTime=update diagram  Latency=0  AutoFrameSizeCalculation=off
      link override ovrdflg: Value=KINP_CANMsgInvalidMETER1_flg_ovrdflg
      link override ovrdval: Value=KINP_CANMsgInvalidMETER1_flg_ovrdval
  bus_creator : BusCreator  Inputs=4
  bus_selector : BusSelector  OutputSignals=VHAL_CANMsgInvalidIVI1_flg,VHAL_CANMsgInvalidIVI2_flg,VHAL_CANMsgInvalidIVIP200_flg,VHAL_CANMsgInvalidMETER1_flg
  not{1..4} (4 alike) : Logic  Operator=NOT  AllPortsSameDT=off  OutDataTypeStr=boolean
  inp_CanValid_bus : Outport
  wires:
  BHAL_outputs/1 -> [BHAL_outputs]
  bus_selector/1 -> CANMsgInvalidIVI1/1  "<VHAL_CANMsgInvalidIVI1_flg>"
  CANMsgInvalidIVI1/1 -> not1/1
  not1/1 -> bus_creator/1  "VINP_CANMsgValidIVI1_flg"
  bus_selector/2 -> CANMsgInvalidIVI2/1  "<VHAL_CANMsgInvalidIVI2_flg>"
  CANMsgInvalidIVI2/1 -> not2/1
  not2/1 -> bus_creator/2  "VINP_CANMsgValidIVI2_flg"
  bus_selector/3 -> CANMsgInvalidIVIP200/1  "<VHAL_CANMsgInvalidIVIP200_flg>"
  CANMsgInvalidIVIP200/1 -> not3/1
  not3/1 -> bus_creator/3  "VINP_CANMsgValidIVIP200_flg"
  bus_selector/4 -> CANMsgInvalidMETER1/1  "<VHAL_CANMsgInvalidMETER1_flg>"
  CANMsgInvalidMETER1/1 -> not4/1
  not4/1 -> bus_creator/4  "VINP_CANMsgValidMETER1_flg"
  [BHAL_outputs] -> bus_selector/1
  bus_creator/1 -> inp_CanValid_bus/1

== system inp/INP/CAN2/CreateBus ==
  inp_CanValid_bus : Inport
  inp_Hal_bus : Inport  Port=2
  UnitConverter_{1..6,8..14,22..25,27..28,33..36,38,41,46,49,52..53,56..61,66..67,72,74..75,78..80,82,84,86..87,89,92..95,98..100,102} (56 alike) : DataTypeConversion  OutDataTypeStr=boolean
  UnitConverter_{7,15,29..32,37,39..40,44..45,47..48,50..51,54..55,69..71,73,83,85,88,90..91,101} (27 alike) : DataTypeConversion  OutDataTypeStr=uint8
  UnitConverter_{16..21,26,42,62..65,68,76..77,81,96..97,103..104} (20 alike) : DataTypeConversion  OutDataTypeStr=single
  UnitConverter_43 : DataTypeConversion  OutDataTypeStr=uint32
  bus_creator : BusCreator  Inputs=104
  bus_selector : BusSelector  OutputSignals=VINP_CANMsgValidIVI1_flg,VINP_CANMsgValidIVI2_flg,VINP_CANMsgValidIVIP200_flg,VINP_CANMsgValidMETER1_flg
  bus_selector_1 : BusSelector  OutputSignals=VINP_AmbLighLowBatAlertSW_flg,VINP_AmbLighSafetyAlertSW_flg,VINP_AmbLightColorSet_enum,VINP_AmbLightDimInDarkSW_flg,VINP_AmbLightSW_flg,VINP_AmbLightWlcmLightSW_flg,VINP_FCPFrEvtBtnACMaxReq_flg,VINP_FCPFrEvtBtnACReq_flg,VINP_FCPFrEvtBtnAutoReq_flg,VINP_FCPFrEvtBtnSyncReq_flg,VINP_IVITimeCheck_enum,VINP_IVITimeDay_DAY,VINP_IVITimeHour_hr,VINP_IVITimeMinute_min,VINP_IVITimeMonth_MONTH,VINP_IVITimeSecond_s,VINP_IVITimeYear_YEAR,VINP_LINKtoDrive_flg,VINP_OpenDrOpenWdoSW_flg,VINP_PWCONTINUEUSE_flg,VINP_SmartEcoModeSW_flg,VINP_ACChgCurSet_A,VINP_AVMErrSTA_flg,VINP_AVMOFFRecButt_flg,VINP_AVMParkingmode_enum,VINP_AVMparkingcancel_enum,VINP_AVMparkingexcute_enum,VINP_CAASSw_enum,VINP_CDLLockButt_flg,VINP_CDLUnlockButt_flg,VINP_DSEATantiset_flg,VINP_DSEATentryfunset_flg,VINP_DSEATventreq_enum,VINP_Distanceunit_flg,VINP_ESCSWCmd_enum,VINP_FSOffSw_enum,VINP_FollowMeSW_flg,VINP_GPSLAT_s,VINP_GPSLONG_enum,VINP_HeadLampSW_enum,VINP_HoodLatchSW_enum,VINP_IVINightModeSta_flg,VINP_IVIPTGModeSW_enum,VINP_IVIPTGStaSW_enum,VINP_IVIPTGUSStaSW_flg,VINP_IVIPWModeReq_enum,VINP_IVIPwrLockSW_enum,VINP_IVIPwroffreq_flg,VINP_IVIRRDefReq_flg,VINP_IVIReqV2L_enum,VINP_IVIScreen_enum,VINP_IVIStartChgreq_flg,VINP_IVIStatus_flg,VINP_IVIStopChgreq_flg,VINP_IVITriggerreq_flg,VINP_IVIUnlockChgreq_flg,VINP_IVIWIMAINSW_flg,VINP_LDrvControlCommand_pct,VINP_LPasControlCommand_pct,VINP_LRLDControlCommand_pct,VINP_LRRDControlCommand_pct,VINP_LightShowStartReq_flg,VINP_LightShowStopReq_flg,VINP_MFRDNBrightReq_pct,VINP_OFFACMODE_enum,VINP_PSEATventreq_enum,VINP_PerdV2L_enum,VINP_RFogLampSW_flg,VINP_RollModeSWCmd_enum,VINP_RoomLampMode_flg,VINP_SOCADJBUTT_flg,VINP_SOCLimitSet_pct,VINP_SOCV2LLimit_pct,VINP_SchedChgStart_flg,VINP_SchedChgStop_flg,VINP_SchedChgbutt_flg,VINP_SchedChglimit_pct,VINP_SchedChgwake_flg,VINP_SenstivityPosition_enum,VINP_SetUnlockSingle_flg,VINP_TCSSWCmd_enum,VINP_TPMSCaliButt_flg,VINP_TPMSResButt_flg,VINP_TurnSwTimeSet_enum,VINP_WalkawayLockSW_flg,VINP_WlcmLightMode_enum,VINP_sigAirIntenZon1Req_enum,VINP_sigDfrstReq_flg,VINP_sigFaceReq_flg,VINP_sigFootReq_flg,VINP_sigRecircReq_flg,VINP_sigSetTempZon1Req_C,VINP_sigSetTempZon2Req_C,VINP_IVIFrAtmoLampCmd_flg,VINP_IVIPassengerdoorSta_flg,VINP_IVIRrAtmoLampCmd_flg,VINP_IVIRrRmLampBrightCmd_enum,VINP_IVIRrRoomlampCmd_flg,VINP_METERKPHCalcu_kph,VINP_ODOMETER_km
  BINP_outputs : Outport
  wires:
  inp_CanValid_bus/1 -> [inp_CanValid_bus]
  inp_Hal_bus/1 -> [inp_Hal_bus]
  bus_selector/1 -> UnitConverter_1/1  "<VINP_CANMsgValidIVI1_flg>"
  UnitConverter_1/1 -> bus_creator/1  "VINP_CANMsgValidIVI1_flg"
  bus_selector/2 -> UnitConverter_2/1  "<VINP_CANMsgValidIVI2_flg>"
  UnitConverter_2/1 -> bus_creator/2  "VINP_CANMsgValidIVI2_flg"
  bus_selector/3 -> UnitConverter_3/1  "<VINP_CANMsgValidIVIP200_flg>"
  UnitConverter_3/1 -> bus_creator/3  "VINP_CANMsgValidIVIP200_flg"
  bus_selector/4 -> UnitConverter_4/1  "<VINP_CANMsgValidMETER1_flg>"
  UnitConverter_4/1 -> bus_creator/4  "VINP_CANMsgValidMETER1_flg"
  bus_selector_1/1 -> UnitConverter_5/1  "<VINP_AmbLighLowBatAlertSW_flg>"
  UnitConverter_5/1 -> bus_creator/5  "VINP_AmbLighLowBatAlertSW_flg"
  bus_selector_1/2 -> UnitConverter_6/1  "<VINP_AmbLighSafetyAlertSW_flg>"
  UnitConverter_6/1 -> bus_creator/6  "VINP_AmbLighSafetyAlertSW_flg"
  bus_selector_1/3 -> UnitConverter_7/1  "<VINP_AmbLightColorSet_enum>"
  UnitConverter_7/1 -> bus_creator/7  "VINP_AmbLightColorSet_enum"
  bus_selector_1/4 -> UnitConverter_8/1  "<VINP_AmbLightDimInDarkSW_flg>"
  UnitConverter_8/1 -> bus_creator/8  "VINP_AmbLightDimInDarkSW_flg"
  bus_selector_1/5 -> UnitConverter_9/1  "<VINP_AmbLightSW_flg>"
  UnitConverter_9/1 -> bus_creator/9  "VINP_AmbLightSW_flg"
  bus_selector_1/6 -> UnitConverter_10/1  "<VINP_AmbLightWlcmLightSW_flg>"
  UnitConverter_10/1 -> bus_creator/10  "VINP_AmbLightWlcmLightSW_flg"
  bus_selector_1/7 -> UnitConverter_11/1  "<VINP_FCPFrEvtBtnACMaxReq_flg>"
  UnitConverter_11/1 -> bus_creator/11  "VINP_FCPFrEvtBtnACMaxReq_flg"
  bus_selector_1/8 -> UnitConverter_12/1  "<VINP_FCPFrEvtBtnACReq_flg>"
  UnitConverter_12/1 -> bus_creator/12  "VINP_FCPFrEvtBtnACReq_flg"
  bus_selector_1/9 -> UnitConverter_13/1  "<VINP_FCPFrEvtBtnAutoReq_flg>"
  UnitConverter_13/1 -> bus_creator/13  "VINP_FCPFrEvtBtnAutoReq_flg"
  bus_selector_1/10 -> UnitConverter_14/1  "<VINP_FCPFrEvtBtnSyncReq_flg>"
  UnitConverter_14/1 -> bus_creator/14  "VINP_FCPFrEvtBtnSyncReq_flg"
  bus_selector_1/11 -> UnitConverter_15/1  "<VINP_IVITimeCheck_enum>"
  UnitConverter_15/1 -> bus_creator/15  "VINP_IVITimeCheck_enum"
  bus_selector_1/12 -> UnitConverter_16/1  "<VINP_IVITimeDay_DAY>"
  UnitConverter_16/1 -> bus_creator/16  "VINP_IVITimeDay_DAY"
  bus_selector_1/13 -> UnitConverter_17/1  "<VINP_IVITimeHour_hr>"
  UnitConverter_17/1 -> bus_creator/17  "VINP_IVITimeHour_hr"
  bus_selector_1/14 -> UnitConverter_18/1  "<VINP_IVITimeMinute_min>"
  UnitConverter_18/1 -> bus_creator/18  "VINP_IVITimeMinute_min"
  bus_selector_1/15 -> UnitConverter_19/1  "<VINP_IVITimeMonth_MONTH>"
  UnitConverter_19/1 -> bus_creator/19  "VINP_IVITimeMonth_MONTH"
  bus_selector_1/16 -> UnitConverter_20/1  "<VINP_IVITimeSecond_s>"
  UnitConverter_20/1 -> bus_creator/20  "VINP_IVITimeSecond_s"
  bus_selector_1/17 -> UnitConverter_21/1  "<VINP_IVITimeYear_YEAR>"
  UnitConverter_21/1 -> bus_creator/21  "VINP_IVITimeYear_YEAR"
  bus_selector_1/18 -> UnitConverter_22/1  "<VINP_LINKtoDrive_flg>"
  UnitConverter_22/1 -> bus_creator/22  "VINP_LINKtoDrive_flg"
  bus_selector_1/19 -> UnitConverter_23/1  "<VINP_OpenDrOpenWdoSW_flg>"
  UnitConverter_23/1 -> bus_creator/23  "VINP_OpenDrOpenWdoSW_flg"
  bus_selector_1/20 -> UnitConverter_24/1  "<VINP_PWCONTINUEUSE_flg>"
  UnitConverter_24/1 -> bus_creator/24  "VINP_PWCONTINUEUSE_flg"
  bus_selector_1/21 -> UnitConverter_25/1  "<VINP_SmartEcoModeSW_flg>"
  UnitConverter_25/1 -> bus_creator/25  "VINP_SmartEcoModeSW_flg"
  bus_selector_1/22 -> UnitConverter_26/1  "<VINP_ACChgCurSet_A>"
  UnitConverter_26/1 -> bus_creator/26  "VINP_ACChgCurSet_A"
  bus_selector_1/23 -> UnitConverter_27/1  "<VINP_AVMErrSTA_flg>"
  UnitConverter_27/1 -> bus_creator/27  "VINP_AVMErrSTA_flg"
  bus_selector_1/24 -> UnitConverter_28/1  "<VINP_AVMOFFRecButt_flg>"
  UnitConverter_28/1 -> bus_creator/28  "VINP_AVMOFFRecButt_flg"
  bus_selector_1/25 -> UnitConverter_29/1  "<VINP_AVMParkingmode_enum>"
  UnitConverter_29/1 -> bus_creator/29  "VINP_AVMParkingmode_enum"
  bus_selector_1/26 -> UnitConverter_30/1  "<VINP_AVMparkingcancel_enum>"
  UnitConverter_30/1 -> bus_creator/30  "VINP_AVMparkingcancel_enum"
  bus_selector_1/27 -> UnitConverter_31/1  "<VINP_AVMparkingexcute_enum>"
  UnitConverter_31/1 -> bus_creator/31  "VINP_AVMparkingexcute_enum"
  bus_selector_1/28 -> UnitConverter_32/1  "<VINP_CAASSw_enum>"
  UnitConverter_32/1 -> bus_creator/32  "VINP_CAASSw_enum"
  bus_selector_1/29 -> UnitConverter_33/1  "<VINP_CDLLockButt_flg>"
  UnitConverter_33/1 -> bus_creator/33  "VINP_CDLLockButt_flg"
  bus_selector_1/30 -> UnitConverter_34/1  "<VINP_CDLUnlockButt_flg>"
  UnitConverter_34/1 -> bus_creator/34  "VINP_CDLUnlockButt_flg"
  bus_selector_1/31 -> UnitConverter_35/1  "<VINP_DSEATantiset_flg>"
  UnitConverter_35/1 -> bus_creator/35  "VINP_DSEATantiset_flg"
  bus_selector_1/32 -> UnitConverter_36/1  "<VINP_DSEATentryfunset_flg>"
  UnitConverter_36/1 -> bus_creator/36  "VINP_DSEATentryfunset_flg"
  bus_selector_1/33 -> UnitConverter_37/1  "<VINP_DSEATventreq_enum>"
  UnitConverter_37/1 -> bus_creator/37  "VINP_DSEATventreq_enum"
  bus_selector_1/34 -> UnitConverter_38/1  "<VINP_Distanceunit_flg>"
  UnitConverter_38/1 -> bus_creator/38  "VINP_Distanceunit_flg"
  bus_selector_1/35 -> UnitConverter_39/1  "<VINP_ESCSWCmd_enum>"
  UnitConverter_39/1 -> bus_creator/39  "VINP_ESCSWCmd_enum"
  bus_selector_1/36 -> UnitConverter_40/1  "<VINP_FSOffSw_enum>"
  UnitConverter_40/1 -> bus_creator/40  "VINP_FSOffSw_enum"
  bus_selector_1/37 -> UnitConverter_41/1  "<VINP_FollowMeSW_flg>"
  UnitConverter_41/1 -> bus_creator/41  "VINP_FollowMeSW_flg"
  bus_selector_1/38 -> UnitConverter_42/1  "<VINP_GPSLAT_s>"
  UnitConverter_42/1 -> bus_creator/42  "VINP_GPSLAT_s"
  bus_selector_1/39 -> UnitConverter_43/1  "<VINP_GPSLONG_enum>"
  UnitConverter_43/1 -> bus_creator/43  "VINP_GPSLONG_enum"
  bus_selector_1/40 -> UnitConverter_44/1  "<VINP_HeadLampSW_enum>"
  UnitConverter_44/1 -> bus_creator/44  "VINP_HeadLampSW_enum"
  bus_selector_1/41 -> UnitConverter_45/1  "<VINP_HoodLatchSW_enum>"
  UnitConverter_45/1 -> bus_creator/45  "VINP_HoodLatchSW_enum"
  bus_selector_1/42 -> UnitConverter_46/1  "<VINP_IVINightModeSta_flg>"
  UnitConverter_46/1 -> bus_creator/46  "VINP_IVINightModeSta_flg"
  bus_selector_1/43 -> UnitConverter_47/1  "<VINP_IVIPTGModeSW_enum>"
  UnitConverter_47/1 -> bus_creator/47  "VINP_IVIPTGModeSW_enum"
  bus_selector_1/44 -> UnitConverter_48/1  "<VINP_IVIPTGStaSW_enum>"
  UnitConverter_48/1 -> bus_creator/48  "VINP_IVIPTGStaSW_enum"
  bus_selector_1/45 -> UnitConverter_49/1  "<VINP_IVIPTGUSStaSW_flg>"
  UnitConverter_49/1 -> bus_creator/49  "VINP_IVIPTGUSStaSW_flg"
  bus_selector_1/46 -> UnitConverter_50/1  "<VINP_IVIPWModeReq_enum>"
  UnitConverter_50/1 -> bus_creator/50  "VINP_IVIPWModeReq_enum"
  bus_selector_1/47 -> UnitConverter_51/1  "<VINP_IVIPwrLockSW_enum>"
  UnitConverter_51/1 -> bus_creator/51  "VINP_IVIPwrLockSW_enum"
  bus_selector_1/48 -> UnitConverter_52/1  "<VINP_IVIPwroffreq_flg>"
  UnitConverter_52/1 -> bus_creator/52  "VINP_IVIPwroffreq_flg"
  bus_selector_1/49 -> UnitConverter_53/1  "<VINP_IVIRRDefReq_flg>"
  UnitConverter_53/1 -> bus_creator/53  "VINP_IVIRRDefReq_flg"
  bus_selector_1/50 -> UnitConverter_54/1  "<VINP_IVIReqV2L_enum>"
  UnitConverter_54/1 -> bus_creator/54  "VINP_IVIReqV2L_enum"
  bus_selector_1/51 -> UnitConverter_55/1  "<VINP_IVIScreen_enum>"
  UnitConverter_55/1 -> bus_creator/55  "VINP_IVIScreen_enum"
  bus_selector_1/52 -> UnitConverter_56/1  "<VINP_IVIStartChgreq_flg>"
  UnitConverter_56/1 -> bus_creator/56  "VINP_IVIStartChgreq_flg"
  bus_selector_1/53 -> UnitConverter_57/1  "<VINP_IVIStatus_flg>"
  UnitConverter_57/1 -> bus_creator/57  "VINP_IVIStatus_flg"
  bus_selector_1/54 -> UnitConverter_58/1  "<VINP_IVIStopChgreq_flg>"
  UnitConverter_58/1 -> bus_creator/58  "VINP_IVIStopChgreq_flg"
  bus_selector_1/55 -> UnitConverter_59/1  "<VINP_IVITriggerreq_flg>"
  UnitConverter_59/1 -> bus_creator/59  "VINP_IVITriggerreq_flg"
  bus_selector_1/56 -> UnitConverter_60/1  "<VINP_IVIUnlockChgreq_flg>"
  UnitConverter_60/1 -> bus_creator/60  "VINP_IVIUnlockChgreq_flg"
  bus_selector_1/57 -> UnitConverter_61/1  "<VINP_IVIWIMAINSW_flg>"
  UnitConverter_61/1 -> bus_creator/61  "VINP_IVIWIMAINSW_flg"
  bus_selector_1/58 -> UnitConverter_62/1  "<VINP_LDrvControlCommand_pct>"
  UnitConverter_62/1 -> bus_creator/62  "VINP_LDrvControlCommand_pct"
  bus_selector_1/59 -> UnitConverter_63/1  "<VINP_LPasControlCommand_pct>"
  UnitConverter_63/1 -> bus_creator/63  "VINP_LPasControlCommand_pct"
  bus_selector_1/60 -> UnitConverter_64/1  "<VINP_LRLDControlCommand_pct>"
  UnitConverter_64/1 -> bus_creator/64  "VINP_LRLDControlCommand_pct"
  bus_selector_1/61 -> UnitConverter_65/1  "<VINP_LRRDControlCommand_pct>"
  UnitConverter_65/1 -> bus_creator/65  "VINP_LRRDControlCommand_pct"
  bus_selector_1/62 -> UnitConverter_66/1  "<VINP_LightShowStartReq_flg>"
  UnitConverter_66/1 -> bus_creator/66  "VINP_LightShowStartReq_flg"
  bus_selector_1/63 -> UnitConverter_67/1  "<VINP_LightShowStopReq_flg>"
  UnitConverter_67/1 -> bus_creator/67  "VINP_LightShowStopReq_flg"
  bus_selector_1/64 -> UnitConverter_68/1  "<VINP_MFRDNBrightReq_pct>"
  UnitConverter_68/1 -> bus_creator/68  "VINP_MFRDNBrightReq_pct"
  bus_selector_1/65 -> UnitConverter_69/1  "<VINP_OFFACMODE_enum>"
  UnitConverter_69/1 -> bus_creator/69  "VINP_OFFACMODE_enum"
  bus_selector_1/66 -> UnitConverter_70/1  "<VINP_PSEATventreq_enum>"
  UnitConverter_70/1 -> bus_creator/70  "VINP_PSEATventreq_enum"
  bus_selector_1/67 -> UnitConverter_71/1  "<VINP_PerdV2L_enum>"
  UnitConverter_71/1 -> bus_creator/71  "VINP_PerdV2L_enum"
  bus_selector_1/68 -> UnitConverter_72/1  "<VINP_RFogLampSW_flg>"
  UnitConverter_72/1 -> bus_creator/72  "VINP_RFogLampSW_flg"
  bus_selector_1/69 -> UnitConverter_73/1  "<VINP_RollModeSWCmd_enum>"
  UnitConverter_73/1 -> bus_creator/73  "VINP_RollModeSWCmd_enum"
  bus_selector_1/70 -> UnitConverter_74/1  "<VINP_RoomLampMode_flg>"
  UnitConverter_74/1 -> bus_creator/74  "VINP_RoomLampMode_flg"
  bus_selector_1/71 -> UnitConverter_75/1  "<VINP_SOCADJBUTT_flg>"
  UnitConverter_75/1 -> bus_creator/75  "VINP_SOCADJBUTT_flg"
  bus_selector_1/72 -> UnitConverter_76/1  "<VINP_SOCLimitSet_pct>"
  UnitConverter_76/1 -> bus_creator/76  "VINP_SOCLimitSet_pct"
  bus_selector_1/73 -> UnitConverter_77/1  "<VINP_SOCV2LLimit_pct>"
  UnitConverter_77/1 -> bus_creator/77  "VINP_SOCV2LLimit_pct"
  bus_selector_1/74 -> UnitConverter_78/1  "<VINP_SchedChgStart_flg>"
  UnitConverter_78/1 -> bus_creator/78  "VINP_SchedChgStart_flg"
  bus_selector_1/75 -> UnitConverter_79/1  "<VINP_SchedChgStop_flg>"
  UnitConverter_79/1 -> bus_creator/79  "VINP_SchedChgStop_flg"
  bus_selector_1/76 -> UnitConverter_80/1  "<VINP_SchedChgbutt_flg>"
  UnitConverter_80/1 -> bus_creator/80  "VINP_SchedChgbutt_flg"
  bus_selector_1/77 -> UnitConverter_81/1  "<VINP_SchedChglimit_pct>"
  UnitConverter_81/1 -> bus_creator/81  "VINP_SchedChglimit_pct"
  bus_selector_1/78 -> UnitConverter_82/1  "<VINP_SchedChgwake_flg>"
  UnitConverter_82/1 -> bus_creator/82  "VINP_SchedChgwake_flg"
  bus_selector_1/79 -> UnitConverter_83/1  "<VINP_SenstivityPosition_enum>"
  UnitConverter_83/1 -> bus_creator/83  "VINP_SenstivityPosition_enum"
  bus_selector_1/80 -> UnitConverter_84/1  "<VINP_SetUnlockSingle_flg>"
  UnitConverter_84/1 -> bus_creator/84  "VINP_SetUnlockSingle_flg"
  bus_selector_1/81 -> UnitConverter_85/1  "<VINP_TCSSWCmd_enum>"
  UnitConverter_85/1 -> bus_creator/85  "VINP_TCSSWCmd_enum"
  bus_selector_1/82 -> UnitConverter_86/1  "<VINP_TPMSCaliButt_flg>"
  UnitConverter_86/1 -> bus_creator/86  "VINP_TPMSCaliButt_flg"
  bus_selector_1/83 -> UnitConverter_87/1  "<VINP_TPMSResButt_flg>"
  UnitConverter_87/1 -> bus_creator/87  "VINP_TPMSResButt_flg"
  bus_selector_1/84 -> UnitConverter_88/1  "<VINP_TurnSwTimeSet_enum>"
  UnitConverter_88/1 -> bus_creator/88  "VINP_TurnSwTimeSet_enum"
  bus_selector_1/85 -> UnitConverter_89/1  "<VINP_WalkawayLockSW_flg>"
  UnitConverter_89/1 -> bus_creator/89  "VINP_WalkawayLockSW_flg"
  bus_selector_1/86 -> UnitConverter_90/1  "<VINP_WlcmLightMode_enum>"
  UnitConverter_90/1 -> bus_creator/90  "VINP_WlcmLightMode_enum"
  bus_selector_1/87 -> UnitConverter_91/1  "<VINP_sigAirIntenZon1Req_enum>"
  UnitConverter_91/1 -> bus_creator/91  "VINP_sigAirIntenZon1Req_enum"
  bus_selector_1/88 -> UnitConverter_92/1  "<VINP_sigDfrstReq_flg>"
  UnitConverter_92/1 -> bus_creator/92  "VINP_sigDfrstReq_flg"
  bus_selector_1/89 -> UnitConverter_93/1  "<VINP_sigFaceReq_flg>"
  UnitConverter_93/1 -> bus_creator/93  "VINP_sigFaceReq_flg"
  bus_selector_1/90 -> UnitConverter_94/1  "<VINP_sigFootReq_flg>"
  UnitConverter_94/1 -> bus_creator/94  "VINP_sigFootReq_flg"
  bus_selector_1/91 -> UnitConverter_95/1  "<VINP_sigRecircReq_flg>"
  UnitConverter_95/1 -> bus_creator/95  "VINP_sigRecircReq_flg"
  bus_selector_1/92 -> UnitConverter_96/1  "<VINP_sigSetTempZon1Req_C>"
  UnitConverter_96/1 -> bus_creator/96  "VINP_sigSetTempZon1Req_C"
  bus_selector_1/93 -> UnitConverter_97/1  "<VINP_sigSetTempZon2Req_C>"
  UnitConverter_97/1 -> bus_creator/97  "VINP_sigSetTempZon2Req_C"
  bus_selector_1/94 -> UnitConverter_98/1  "<VINP_IVIFrAtmoLampCmd_flg>"
  UnitConverter_98/1 -> bus_creator/98  "VINP_IVIFrAtmoLampCmd_flg"
  bus_selector_1/95 -> UnitConverter_99/1  "<VINP_IVIPassengerdoorSta_flg>"
  UnitConverter_99/1 -> bus_creator/99  "VINP_IVIPassengerdoorSta_flg"
  bus_selector_1/96 -> UnitConverter_100/1  "<VINP_IVIRrAtmoLampCmd_flg>"
  UnitConverter_100/1 -> bus_creator/100  "VINP_IVIRrAtmoLampCmd_flg"
  bus_selector_1/97 -> UnitConverter_101/1  "<VINP_IVIRrRmLampBrightCmd_enum>"
  UnitConverter_101/1 -> bus_creator/101  "VINP_IVIRrRmLampBrightCmd_enum"
  bus_selector_1/98 -> UnitConverter_102/1  "<VINP_IVIRrRoomlampCmd_flg>"
  UnitConverter_102/1 -> bus_creator/102  "VINP_IVIRrRoomlampCmd_flg"
  bus_selector_1/99 -> UnitConverter_103/1  "<VINP_METERKPHCalcu_kph>"
  UnitConverter_103/1 -> bus_creator/103  "VINP_METERKPHCalcu_kph"
  bus_selector_1/100 -> UnitConverter_104/1  "<VINP_ODOMETER_km>"
  UnitConverter_104/1 -> bus_creator/104  "VINP_ODOMETER_km"
  [inp_CanValid_bus] -> bus_selector/1
  [inp_Hal_bus] -> bus_selector_1/1
  bus_creator/1 -> BINP_outputs/1
